simulink model "TLE9879_MAVlink"  (R2021b)
settings: Solver=FixedStepAuto  StartTime=0.0  StopTime=inf  RelTol=1e-3
libraries: instrumentseriallib x3, uavmavlinklib x3
settings Model: Creator=shun  LastModifiedBy=shun

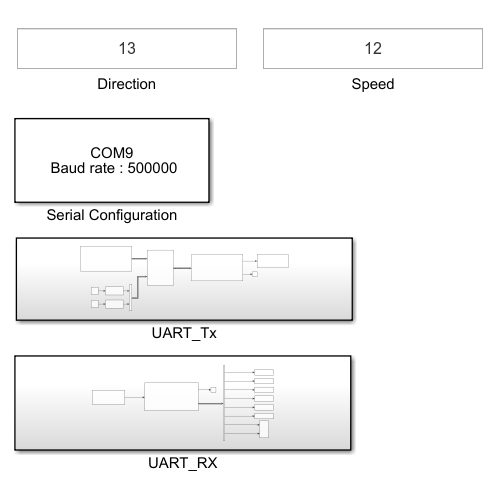
[thumbnail: Simulink's stored preview of the top-level diagram]
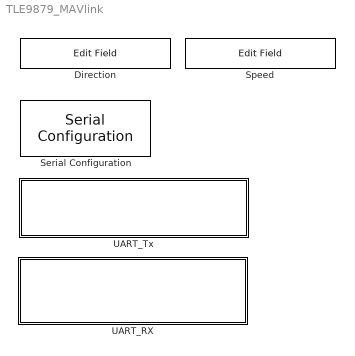
== system TLE9879_MAVlink ==
  Direction : EditField  LabelPosition=Hide  ShowInitialText=on  Alignment=Center
  Serial Configuration : instrumentseriallib/Serial Configuration  Priority=-200000  Port=COM9  ComPort=COM9  BaudRate=500000  DataBits=8  Parity=none  StopBits=1  ByteOrder=little-endian  FlowControl=none  Timeout=0.01  SimulateUsing=Interpreted execution  BlockInModel=on
  Speed : EditField  LabelPosition=Hide  ShowInitialText=on  Alignment=Center
  UART_RX : Subsystem
  UART_Tx : Subsystem

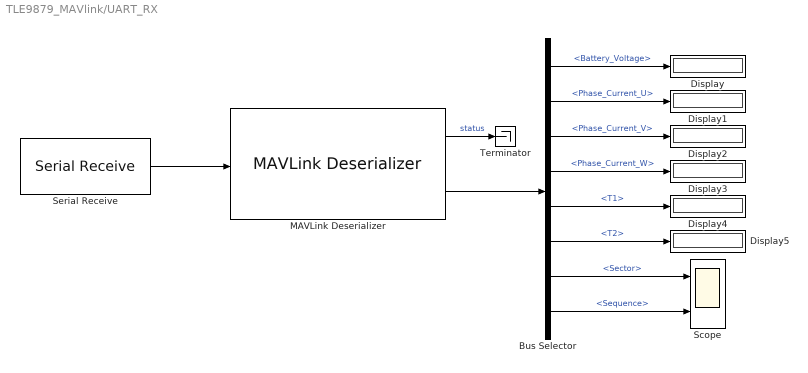
== system TLE9879_MAVlink/UART_RX ==
  Bus Selector : BusSelector  OutputSignals=Payload.Battery_Voltage,Payload.Phase_Current_U,Payload.Phase_Current_V,Payload.Phase_Current_W,Payload.T1,Payload.T2,Payload.Sector,Sequence
  Display{,1..5} (6 alike) : Display
  MAVLink Deserializer : uavmavlinklib/MAVLink Deserializer  dialectSource=Specify your own  dialect=common.xml  dialectCustom=D:\Mavlink\TLE9879_Mavlink\TLE9879_MAVlink.xml  version=1  messageType=PMSM_Status  inputDataLength=off  SystemIDFilter=off  systemID=1  ComponentIDFilter=off  componentID=1  queueMsg=off  queueMsgSize=50  dropNum=off
      settings: SourceProductBaseCode=UV
  Scope : Scope  NumInputPorts=2
  Serial Receive : instrumentseriallib/Serial Receive  Priority=1  Port=COM9  ComPort=COM9  DataType=uint8  SaveDataType=uint8  ToggleHeader=off  Header=[]  ToggleTerminator=off  Terminator=<none>  CustomTerminator=[]  ToggleDataSize=on  DataSize=[1 1]  EnableBlockingMode=on  ActionDataUnavailable=Output last received value  ActionWhenDataUnavailable=Output last received value  CustomValue=0  SampleTime=0.01  SimulateUsing=Interpreted execution  BlockInModel=on
  Terminator : Terminator
  wires:
  Bus Selector/4 -> Display3/1  "<Phase_Current_W>"
  Bus Selector/7 -> Scope/1  "<Sector>"
  Bus Selector/3 -> Display2/1  "<Phase_Current_V>"
  MAVLink Deserializer/1 -> Terminator/1  "status"
  Serial Receive/1 -> MAVLink Deserializer/1
  Bus Selector/8 -> Scope/2  "<Sequence>"
  MAVLink Deserializer/2 -> Bus Selector/1
  Bus Selector/1 -> Display/1  "<Battery_Voltage>"
  Bus Selector/2 -> Display1/1  "<Phase_Current_U>"
  Bus Selector/6 -> Display5/1  "<T2>"
  Bus Selector/5 -> Display4/1  "<T1>"

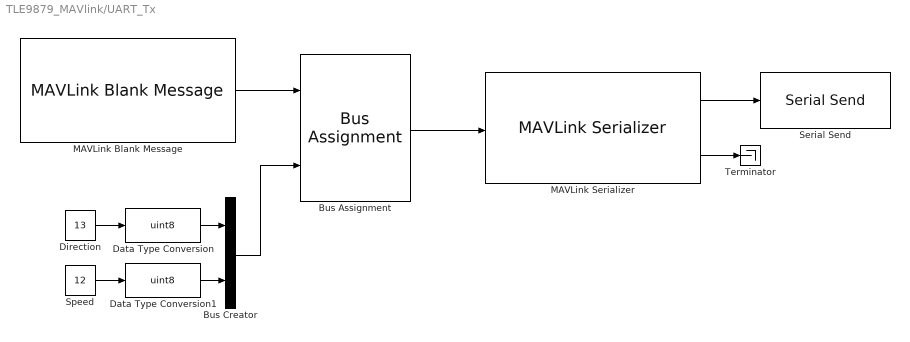
== system TLE9879_MAVlink/UART_Tx ==
  Bus Assignment : BusAssignment  AssignedSignals=Payload
  Bus Creator : BusCreator  Inputs=2
  Data Type Conversion : DataTypeConversion  OutDataTypeStr=uint8
  Data Type Conversion1 : DataTypeConversion  OutDataTypeStr=uint8
  Direction : Constant  Value=13
  MAVLink Blank Message : uavmavlinklib/MAVLink Blank Message  dialectSource=Specify your own  dialect=common.xml  dialectCustom=D:\Mavlink\TLE9879_Mavlink\TLE9879_MAVlink.xml  version=1  messageType=PMSM_Command  SystemID=1  ComponentID=1  SampleTime=1
      settings: SourceProductBaseCode=UV
  MAVLink Serializer : uavmavlinklib/MAVLink Serializer  dialectSource=Specify your own  dialect=common.xml  dialectCustom=D:\Mavlink\TLE9879_Mavlink\TLE9879_MAVlink.xml  version=1  messageType=PMSM_Command
      settings: SourceProductBaseCode=UV
  Serial Send : instrumentseriallib/Serial Send  Priority=1  Port=COM9  ComPort=COM9  Header=[]  Terminator=<none>  CustomTerminator=[]  EnableBlockingMode=on  SimulateUsing=Interpreted execution  BlockInModel=on
  Speed : Constant  Value=12
  Terminator : Terminator
  wires:
  Data Type Conversion1/1 -> Bus Creator/2
  Speed/1 -> Data Type Conversion1/1
  Bus Creator/1 -> Bus Assignment/2
  MAVLink Serializer/2 -> Terminator/1
  Direction/1 -> Data Type Conversion/1
  MAVLink Serializer/1 -> Serial Send/1
  Data Type Conversion/1 -> Bus Creator/1
  MAVLink Blank Message/1 -> Bus Assignment/1
  Bus Assignment/1 -> MAVLink Serializer/1
